simulink library "lib"  (R2014b)
settings: Solver=ode45  StartTime=0.0  StopTime=10.0  RelTol=1e-3
undefined symbols (not defined in the file): avoidPointFnc, calcTauGravFnc, dim, T0, Tf
libraries: simulink x3
settings Model: Creator=Edoardo  LastModifiedBy=Edoardo

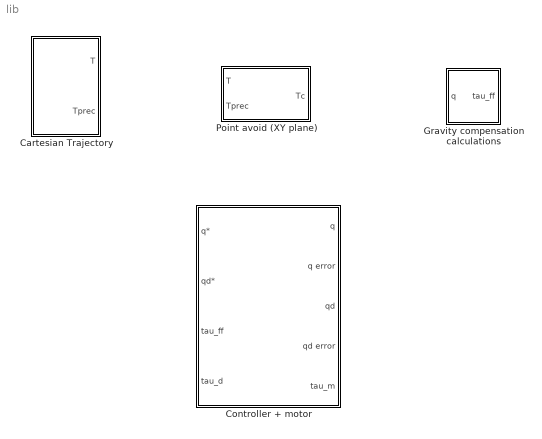
== system lib ==
  Cartesian Trajectory : Subsystem  mask(Cartesian trajectory planner){ref=Internal, T0=T0, Tf=Tf, v={}, Tmax=30, Ts=0.1, rot_type=Quaternions}
      mask prompts: ref "Reference"; T0 "Init. pose"; Tf "Final pose"; v "Vias"; Tmax "Tmax (s)"; Ts "Ts (s)"; rot_type "Rotation type"
      mask help:
      | Plans the trajectory between two poses following a straight trajectory.
      | Orientation is planned with one of the 3 available procedures.
      mask init:
      | % Check if input data is correct
      | assert(iscell(v),'Not a cell');
      | assert(Tmax>0,'Tmax must be greater than 0');
      | assert(Ts>0,'Ts must be greater than 0');
      | 
      | % If wanted to implement External/Internal reference, look at the example
      | % of dynamical changes of masks
      | 
      | % Calculate trajectory
      | n = Tmax/Ts + 1;
      | viasNum = length(v) + 1; % Considers Tf as via
      | 
      | n2 = floor(n/viasNum);
      | 
      | vias{1} = T0;
      | vias = cat(2,vias,v);
      | vias{end+1} = Tf;
      | 
      | T = T0;
      | for i=1:viasNum
      |     if i == viasNum
      |         n2 = n - n2*(viasNum-1);
      |     end
      |     Tx = ctraj(vias{i},vias{i+1},n2);
      |     T = cat(3,T,Tx);
      | end
      | T(:,:,1) = [];
      mask Help: Help
      mask TypeOptions ref: Internal | External
      mask Callback ref:
      | % Get parameters from 'ref' prompt
      | ref = get_param(gcb,'ref');
      | maskEnab = get_param(gcb,'MaskEnables');
      | 
      | % Change enables based on choice on 'ref' prompt
      | if strcmp(ref,'Internal')
      |     maskEnab{2} = 'on';
      |     maskEnab{3} = 'on';
      |     maskEnab{4} = 'on';
      |     maskEnab{5} = 'on';
      |     set_param(gcb,'MaskEnables',maskEnab);
      | else
      |     maskEnab{2} = 'off';
      |     maskEnab{3} = 'off';
      |     maskEnab{4} = 'off';
      |     maskEnab{5} = 'off';
      |     set_param(gcb,'MaskEnables',maskEnab);
      | end
      mask TypeOptions rot_type: Euler | Planar sliding | Quaternions
  Controller + motor : Subsystem  mask{Kt=0.228, tau_max=0.9, Jm=200e-6, Jl=2, G=100, B=817e-6, omega_max=165, Kp_v=1, Ki_v=5, Kd_v=0, Kp_p=20, Ki_p=0, Kd_p=0, Kff_p=0, Ts=0.001}
      mask prompts: Kt "Motor torque constant (Kt) [Nm/A]"; tau_max "Max torque (tau_max) [Nm]"; Jm "Motor shaft inertia (Jm) [kg*m^2]"; Jl "Load inertia (Jl) [kg*m^2]"; G "Gearbox transformation ratio (G)"; B "Motor viscous friction (B) [Nm*s/rad]"; omega_max "Max speed (omega_max) [rad/s]"; Kp_v "Proportional gain (Kp)"; Ki_v "Integral gain (Ki)"; Kd_v "Derivative gain (Kd)"; Kp_p "Proportional gain (Kp)"; Ki_p "Integral gain (Ki)"; Kd_p "Derivative gain (Kd)"; Kff_p "Feedforward gain (Kff)"; Ts "Sample time (Ts)"
      mask DialogControl Container7 Prompt: Velocity loop
      mask DialogControl Container9 Prompt: Position loop
  Gravity compensation calculations : Subsystem
  Point avoid (XY plane) : Subsystem  mask{pt=[0 0 0], r=0.1}
      mask prompts: pt "Point"; r "Radius"

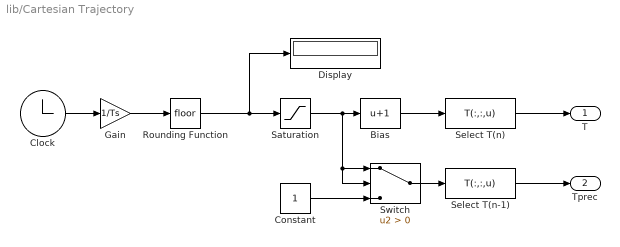
== system lib/Cartesian Trajectory ==
  Bias : Bias  Bias=1
  Clock : Clock
  Constant : Constant
  Display : Display
  Gain : Gain  Gain=1/Ts
  Rounding Function : Rounding
  Saturation : Saturate  UpperLimit=Tmax/Ts
  Select T(n) : MATLABFcn  MATLABFcn=T(:,:,u)  OutputDimensions=[4 4]  Output1D=off
  Select T(n-1) : MATLABFcn  MATLABFcn=T(:,:,u)  OutputDimensions=[4 4]  Output1D=off
  Switch : Switch  Criteria=u2 > Threshold
  T : Outport
  Tprec : Outport  Port=2
  wires:
  Clock/1 -> Gain/1
  Select T(n)/1 -> T/1
  Gain/1 -> Rounding Function/1
  Rounding Function/1 -> Display/1, Saturation/1
  Saturation/1 -> Switch/2, Switch/1, Bias/1
  Bias/1 -> Select T(n)/1
  Select T(n-1)/1 -> Tprec/1
  Constant/1 -> Switch/3
  Switch/1 -> Select T(n-1)/1

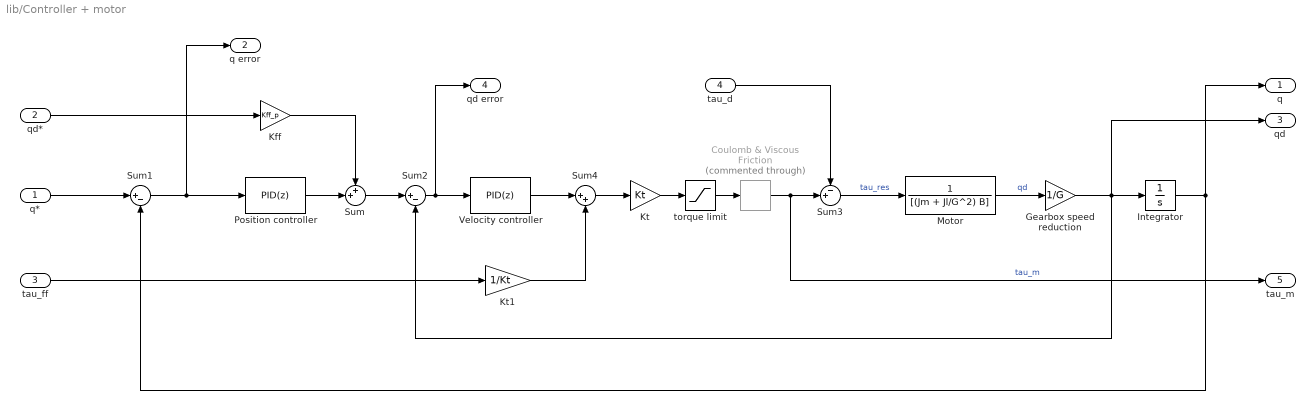
== system lib/Controller + motor ==
  q* : Inport
  qd* : Inport  Port=2
  tau_ff : Inport  Port=3
  tau_d : Inport  Port=4
  Coulomb & Viscous Friction : simulink/Discontinuities/Coulomb & Viscous Friction  Commented=through  offset=0.126  gain=1
  Gearbox speed reduction : Gain  Gain=1/G
  Integrator : Integrator
  Kff : Gain  Gain=Kff_p
  Kt : Gain  Gain=Kt
  Kt1 : Gain  Gain=1/Kt
  Motor : TransferFcn  Denominator=[(Jm + Jl/G^2) B]  ContinuousStateAttributes='qd'
  Position controller : simulink/Continuous/PID Controller  Controller=PID  TimeDomain=Discrete-time  SampleTime=Ts  IntegratorMethod=Forward Euler  FilterMethod=Forward Euler  Form=Parallel  P=Kp_p  I=Ki_p  D=Kd_p  N=100  InitialConditionSource=internal  InitialConditionForIntegrator=0  InitialConditionForFilter=0  ExternalReset=none  LimitOutput=off  UpperSaturationLimit=1  LowerSaturationLimit=-1  LinearizeAsGain=on  AntiWindupMode=none  Kb=1  TrackingMode=off  Kt=1  PParamMin=[]  PParamMax=[]  IParamMin=[]  IParamMax=[]  DParamMin=[]  DParamMax=[]  NParamMin=[]  NParamMax=[]  KbParamMin=[]  KbParamMax=[]  KtParamMin=[]  KtParamMax=[]  POutMin=[]  POutMax=[]  IOutMin=[]  IOutMax=[]  DOutMin=[]  DOutMax=[]  NOutMin=[]  NOutMax=[]  KbOutMin=[]  KbOutMax=[]  KtOutMin=[]  KtOutMax=[]  IntegratorOutMin=[]  IntegratorOutMax=[]  FilterOutMin=[]  FilterOutMax=[]  SumOutMin=[]  SumOutMax=[]  SumI1OutMin=[]  SumI1OutMax=[]  SumI2OutMin=[]  SumI2OutMax=[]  SumI3OutMin=[]  SumI3OutMax=[]  SumDOutMin=[]  SumDOutMax=[]  SaturationOutMin=[]  SaturationOutMax=[]  IntegratorContinuousStateAttributes=''  IntegratorStateMustResolveToSignalObject=off  IntegratorRTWStateStorageClass=Auto  FilterContinuousStateAttributes=''  FilterStateMustResolveToSignalObject=off  FilterRTWStateStorageClass=Auto  DifferentiatorICPrevScaledInput=0  DifferentiatorOutMin=[]  DifferentiatorOutMax=[]  UseFilter=on
  Sum : Sum  Inputs=++|
  Sum1 : Sum  Inputs=|+-
  Sum2 : Sum  Inputs=|+-
  Sum3 : Sum  Inputs=-+|
  Sum4 : Sum  Inputs=|++
  Velocity controller : simulink/Continuous/PID Controller  Controller=PID  TimeDomain=Discrete-time  SampleTime=Ts  IntegratorMethod=Forward Euler  FilterMethod=Forward Euler  Form=Parallel  P=Kp_v  I=Ki_v  D=Kd_v  N=100  InitialConditionSource=internal  InitialConditionForIntegrator=0  InitialConditionForFilter=0  ExternalReset=none  LimitOutput=off  UpperSaturationLimit=1  LowerSaturationLimit=-1  LinearizeAsGain=on  AntiWindupMode=none  Kb=1  TrackingMode=off  Kt=1  PParamMin=[]  PParamMax=[]  IParamMin=[]  IParamMax=[]  DParamMin=[]  DParamMax=[]  NParamMin=[]  NParamMax=[]  KbParamMin=[]  KbParamMax=[]  KtParamMin=[]  KtParamMax=[]  POutMin=[]  POutMax=[]  IOutMin=[]  IOutMax=[]  DOutMin=[]  DOutMax=[]  NOutMin=[]  NOutMax=[]  KbOutMin=[]  KbOutMax=[]  KtOutMin=[]  KtOutMax=[]  IntegratorOutMin=[]  IntegratorOutMax=[]  FilterOutMin=[]  FilterOutMax=[]  SumOutMin=[]  SumOutMax=[]  SumI1OutMin=[]  SumI1OutMax=[]  SumI2OutMin=[]  SumI2OutMax=[]  SumI3OutMin=[]  SumI3OutMax=[]  SumDOutMin=[]  SumDOutMax=[]  SaturationOutMin=[]  SaturationOutMax=[]  IntegratorContinuousStateAttributes=''  IntegratorStateMustResolveToSignalObject=off  IntegratorRTWStateStorageClass=Auto  FilterContinuousStateAttributes=''  FilterStateMustResolveToSignalObject=off  FilterRTWStateStorageClass=Auto  DifferentiatorICPrevScaledInput=0  DifferentiatorOutMin=[]  DifferentiatorOutMax=[]  UseFilter=on
  torque limit : Saturate  UpperLimit=tau_max  LowerLimit=-tau_max
  q : Outport
  q error : Outport  Port=2
  qd : Outport  Port=3
  qd error : Outport  Port=4
  tau_m : Outport  Port=5
  wires:
  Sum1/1 -> Position controller/1, q error/1
  q*/1 -> Sum1/1
  Integrator/1 -> Sum1/2, q/1
  Sum/1 -> Sum2/1
  Sum3/1 -> Motor/1  "tau_res"
  Sum2/1 -> Velocity controller/1, qd error/1
  Motor/1 -> Gearbox speed reduction/1  "qd"
  tau_d/1 -> Sum3/1
  torque limit/1 -> Coulomb & Viscous Friction/1
  qd*/1 -> Kff/1
  Kt/1 -> torque limit/1
  Velocity controller/1 -> Sum4/1
  Sum4/1 -> Kt/1
  tau_ff/1 -> Kt1/1
  Kt1/1 -> Sum4/2
  Kff/1 -> Sum/1
  Position controller/1 -> Sum/2
  Coulomb & Viscous Friction/1 -> Sum3/2, tau_m/1  "tau_m"
  Gearbox speed reduction/1 -> Sum2/2, qd/1, Integrator/1

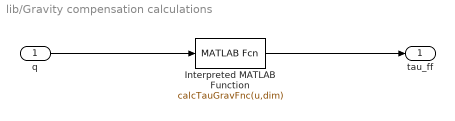
== system lib/Gravity compensation calculations ==
  q : Inport
  Interpreted MATLAB Function : MATLABFcn  MATLABFcn=calcTauGravFnc(u,dim)  OutputDimensions=6  Output1D=off
  tau_ff : Outport
  wires:
  q/1 -> Interpreted MATLAB Function/1
  Interpreted MATLAB Function/1 -> tau_ff/1

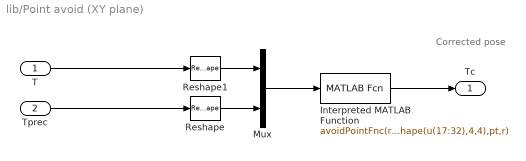
== system lib/Point avoid (XY plane) ==
  note: Corrected pose
  T : Inport
  Tprec : Inport  Port=2
  Interpreted MATLAB Function : MATLABFcn  MATLABFcn=avoidPointFnc(reshape(u(1:16),4,4),reshape(u(17:32),4,4),pt,r)  OutputDimensions=[4 4]  Output1D=off
  Mux : Mux  Inputs=2
  Reshape : Reshape  OutputDimensions=1
  Reshape1 : Reshape  OutputDimensions=1
  Tc : Outport
  wires:
  Interpreted MATLAB Function/1 -> Tc/1
  T/1 -> Reshape1/1
  Mux/1 -> Interpreted MATLAB Function/1
  Reshape1/1 -> Mux/1
  Reshape/1 -> Mux/2
  Tprec/1 -> Reshape/1
